simulink model "tp5_5_emetteur_template_usrp"  (R2023a)
settings: Solver=FixedStepDiscrete  StartTime=0.0  StopTime=inf  RelTol=1e-3
PreLoadFcn:
  | T_s_short=160e-6;
  | N=36;
  | N_IFFT=64;
  | T_e = T_s_short/N_IFFT;
  | f_e=1/T_e;
  | 
  | 
  | %% nombre d'éléments nuls à ajouter au vecteur X, resp avant et après les N ss porteuses actives
  | Z_d=ceil((N_IFFT-N)/2);
  | Z_u=floor((N_IFFT-N)/2);
  | 
  | %% taille du préfixe cyclique et temps symbole rallongé
  | v=8;
  | T_s=(N_IFFT+v)*T_e;
  | 
  | %% pilotes
  | r=0.25;
  | 
  | %% la trame
  | t=10;
  | T_t=t*T_s;
  | 
  | %% le codage binaire du message
  | capa_symbole = N*(1-r)*2;
  | str='coucou';
  | message=double(dec2bin(str,8)=='1');% zeros(6-strlength(str),8)];
  | assert(capa_symbole > numel(message), 'message trop long');
  | message_pad=capa_symbole-numel(message);
InitFcn:
  | T_s_short=160e-6;
  | N=36;
  | N_IFFT=64;
  | T_e = T_s_short/N_IFFT;
  | f_e=1/T_e;
  | 
  | 
  | %% nombre d'éléments nuls à ajouter au vecteur X, resp avant et après les N ss porteuses actives
  | Z_d=ceil((N_IFFT-N)/2);
  | Z_u=floor((N_IFFT-N)/2);
  | 
  | %% taille du préfixe cyclique et temps symbole rallongé
  | v=8;
  | T_s=(N_IFFT+v)*T_e;
  | 
  | %% pilotes
  | r=0.25;
  | 
  | %% la trame
  | t=10;
  | T_t=t*T_s;
  | 
  | %% le codage binaire du message
  | capa_symbole = N*(1-r)*2;
  | str='coucou';
  | message=double(dec2bin(str,8)=='1');% zeros(6-strlength(str),8)];
  | assert(capa_symbole > numel(message), 'message trop long');
  | message_pad=capa_symbole-numel(message);
libraries: dspindex x3, commseqgen3 x2, commutil2 x2, commrandsrc3 x1, dspxfrm3 x1, commdigbbndpm3 x1, commsdrhw_v2 x1
Description:
  | This model uses Universal Software Radio Peripheral (USRP) hardware with Simulink(R) to perform FM demodulation and stereo decoding.
settings Model: SimulationMode=accelerator  Creator=speychet  LastModifiedBy=pjoseph
settings SolverCC: AlgebraicLoopSolver=TrustRegion
settings DataIOCC: SaveFormat=Structure  SaveOutput=off  SignalLogging=off  DSMLogging=off  SaveTime=off  ReturnWorkspaceOutputs=off
settings OptimizationCC: ExpressionDepthLimit=2147483647  EfficientMapNaN2IntZero=off  LifeSpan=inf  SimCompilerOptimization=on
settings DebuggingCC: UnderspecifiedInitializationDetection=Classic  MergeDetectMultiDrivingBlocksExec=none  SolverPrmCheckMsg=warning  InheritedTsInSrcMsg=none  MultiTaskCondExecSysMsg=none  ParameterPrecisionLossMsg=none  FcnCallInpInsideContextMsg=warning  UnconnectedInputMsg=warning  UnconnectedOutputMsg=warning  UnconnectedLineMsg=warning  AllowSymbolicDim=off  StateNameClashWarn=warning  SFUnexpectedBacktrackingDiag=warning  SFNoUnconditionalDefaultTransitionDiag=warning  SFExecutionAtInitializationDiag=none  ArithmeticOperatorsInVariantConditions=warning
settings HardwareCC: ProdBitPerPointer=32  ProdBitPerSizeT=32  ProdBitPerPtrDiffT=32  ProdLargestAtomicFloat=None  ProdIntDivRoundTo=Undefined  ProdEndianess=Unspecified  ProdWordSize=32  ProdHWDeviceType=32-bit Generic  TargetBitPerPointer=64  TargetBitPerSizeT=64  TargetBitPerPtrDiffT=64  TargetLongLongMode=on  TargetIntDivRoundTo=Zero  TargetEndianess=LittleEndian  TargetWordSize=64  TargetHWDeviceType=Generic->MATLAB Host Computer  ProdEqTarget=off
settings ModelReferenceCC: EnableRefExpFcnMdlSchedulingChecks=on  PropagateSignalLabelsOutOfModel=off
settings SFSimCC: SimIntegrity=off  SimUseLocalCustomCode=off  CustomCodeUndefinedFunction=UseInterfaceOnly
settings RTWCC: RTWUseLocalCustomCode=off
settings RTWCC: CustomSourceCode=|
  | #include <stdio.h>
  | #include <stdlib.h>
settings CodeAppCC: MaxIdLength=128  StateflowObjectComments=on
settings GRTTargetCC: TargetLangStandard=C89/C90 (ANSI)  CombineOutputUpdateFcns=off  GRTInterface=on
settings ConfigComp: CovMetricSettings=dw  CovSaveCumulativeToWorkspaceVar=on  CovSaveSingleToWorkspaceVar=on  CovExternalEMLEnable=off  CovSFcnEnable=off

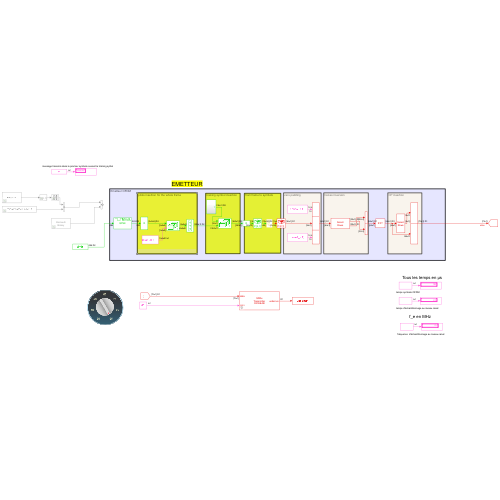
[thumbnail: Simulink's stored preview of the top-level diagram]
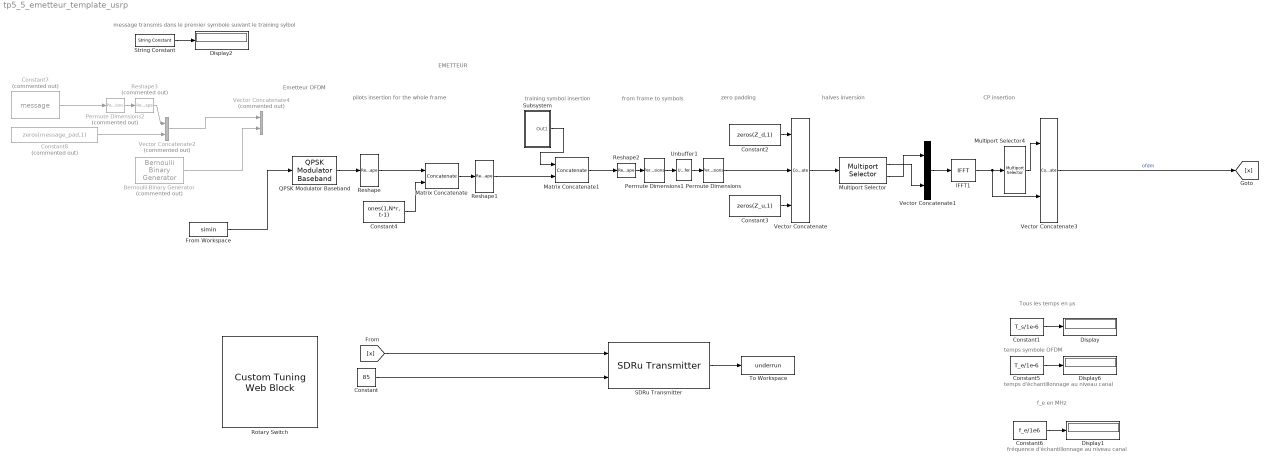
== system tp5_5_emetteur_template_usrp ==
  note: temps symbole OFDM
  note: fréquence d'échantillonnage au niveau canal
  note: CP insertion
  note: temps d'échantillonnage au niveau canal
  note: Tous les temps en µs
  note: pilots insertion for the whole frame
  note: halves inversion
  note: f_e en MHz
  note: zero padding
  note: Emetteur OFDM
  note: EMETTEUR
  note: training symbol insertion
  note: message transmis dans le premier symbole suivant le training sylbol
  note: from frame to symbols
  Bernoulli Binary Generator : commrandsrc3/Bernoulli Binary Generator  Commented=on  ProbabilityOfZero=0.5  SeedSource=Auto  Seed=0  SampleTime=T_t/((t-2)*N*(1-r)*2)  SamplesPerFrame=(t-2)*N*(1-r)*2  OutputDataType=double  SimulateUsing=Code generation
  Constant : Constant  Value=85
  Constant1 : Constant  Value=T_s/1e-6
  Constant2 : Constant  Value=zeros(Z_d,1)
  Constant3 : Constant  Value=zeros(Z_u,1)
  Constant4 : Constant  Value=ones(1,N*r, t-1)  VectorParams1D=off
  Constant5 : Constant  Value=T_e/1e-6
  Constant6 : Constant  Value=f_e/1e6
  Constant7 : Constant  Commented=on  Value=message
  Constant8 : Constant  Commented=on  Value=zeros(message_pad,1)  VectorParams1D=off
  Display{,1..2,6} (4 alike) : Display
  From Workspace : FromWorkspace  VariableName=simin  OutDataTypeStr=double  SampleTime=T_t  Interpolate=off  OutputAfterFinalValue=Holding final value
  IFFT1 : dspxfrm3/IFFT  FFTImplementation=Auto  CompMethod=Table lookup  TableOpt=NEW  TableOptActive=Speed  BitRevOrder=off  cs_in=off  Normalize=on  InheritFFTLength=on  FFTLength=64  WrapInput=on  mode=Complex  outSamplingMode=Sample based  roundingMode=Floor  overflowMode=off  firstCoeffDataTypeStr=Inherit: Same word length as input  firstCoeffLastDataTypeStr=Inherit: Same word length as input  outputMin=[]  outputMax=[]
  Matrix Concatenate : Concatenate  Mode=Multidimensional array
  Matrix Concatenate1 : Concatenate  Mode=Multidimensional array
  Multiport Selector : dspindex/Multiport Selector  rowsOrCols=Rows  idxCellArray={ [1:N_IFFT/2], [N_IFFT/2+1:N_IFFT] }  idxErrMode=Clip Index
  Multiport Selector4 : dspindex/Multiport Selector  rowsOrCols=Rows  idxCellArray={[N_IFFT-v+1:N_IFFT]}  idxErrMode=Clip Index
  Permute Dimensions : PermuteDimensions
  Permute Dimensions1 : PermuteDimensions
  Permute Dimensions2 : PermuteDimensions  Commented=on
  QPSK Modulator Baseband : commdigbbndpm3/QPSK Modulator Baseband  InType=Bit  Enc=Gray  Ph=pi/4  outDtype=double  outWordLen=16  outUDDataType=sfix(16)  outFracLenMode=Best precision  outFracLen=15  outDataTypeStr=double  outLastDataTypeStr=double
  Reshape : Reshape  OutputDimensionality=Customize  OutputDimensions=[(1-r)/r,N*r, t-1]
  Reshape1 : Reshape  OutputDimensionality=Column vector (2-D)
  Reshape2 : Reshape  OutputDimensionality=Customize  OutputDimensions=[N,t]
  Reshape3 : Reshape  Commented=on  OutputDimensionality=Column vector (2-D)
  Rotary Switch : CustomTuningWebBlock  LabelPosition=Hide  ShowInitialText=on  Configuration="{\"components\":[{\"name\":\"RotarySwitchComponent\",\"settings\":{\"arcAngle\":300,\"arcAngleOffset\":120,\"handle\":{\"size\":[150,150],\"src\":\"data:image\\/svg+xml;base64,PHN2ZyBpZD0iTGF5ZXJfMSIgZGF0YS1uYW1lPSJMYXllciAxIiB4bWxucz0iaHR0cDovL3d3dy53My5vcmcvMjAwMC9zdmciIHhtbG5zOnhsaW5rPSJodHRwOi8vd3d3LnczLm9yZy8xOTk5L3hsaW5rIiB2aWV3Qm94PSIwIDAgMTIxIDEyMSI+PGRlZnM+PHN0eWxlPi5jbHMtMXtmaWxsOnVybCgjbGluZWFyLWdyYWRpZW50KTt9LmNscy0yLC5jbHMtM3tmaWxsOiNkMWQxZDE7fS5jbHMtM3tzdHJva2U6I2I3YjdiNztzdHJva2UtbWl0ZXJsaW1pdDoxMDtzdHJva2Utd2lkdGg6MC4yNXB4O30uY2xzLTR7ZmlsbDojZjMwMDAwO30uY2xzLTV7ZmlsbDojZjIxNzY3O308L3N0eWxlPjxsaW5lYXJHcmFkaWVudCBpZD0ibGluZWFyLWdyYWRpZW50IiB4MT0iNjAuNSIgeTE9IjEyMC41IiB4Mj0iNjAuNSIgeTI9IjAuNSIgZ3JhZGllbnRVbml0cz0idXNlclNwYWNlT25Vc2UiPjxzdG9wIG9mZnNldD0iMCIgc3RvcC1jb2xvcj0iI2QxZDFkMSIvPjxzdG9wIG9mZnNldD0iMC4xIiBzdG9wLWNvbG9yPSIjY2VjZWNlIi8+PHN0b3Agb2Zmc2V0PSIwLjE5IiBzdG9wLWNvbG9yPSIjYzNjM2MzIi8+PHN0b3Agb2Zmc2V0PSIwLjI4IiBzdG9wLWNvbG9yPSIjYjFiMWIxIi8+PHN0b3Agb2Zmc2V0PSIwLjM2IiBzdG9wLWNvbG9yPSIjOTg5ODk4Ii8+PHN0b3Agb2Zmc2V0PSIwLjQ0IiBzdG9wLWNvbG9yPSIjNzg3ODc4Ii8+PHN0b3Agb2Zmc2V0PSIwLjQ2IiBzdG9wLWNvbG9yPSIjNmI2YjZiIi8+PHN0b3Agb2Zmc2V0PSIwLjU0IiBzdG9wLWNvbG9yPSIjNmI2YjZiIi8+PHN0b3Agb2Zmc2V0PSIwLjU2IiBzdG9wLWNvbG9yPSIjNzY3Njc2Ii8+PHN0b3Agb2Zmc2V0PSIwLjY0IiBzdG9wLWNvbG9yPSIjOTc5Nzk3Ii8+PHN0b3Agb2Zmc2V0PSIwLjcyIiBzdG9wLWNvbG9yPSIjYjBiMGIwIi8+PHN0b3Agb2Zmc2V0PSIwLjgxIiBzdG9wLWNvbG9yPSIjYzNjM2MzIi8+PHN0b3Agb2Zmc2V0PSIwLjkiIHN0b3AtY29sb3I9IiNjZGNkY2QiLz48c3RvcCBvZmZzZXQ9IjEiIHN0b3AtY29sb3I9IiNkMWQxZDEiLz48L2xpbmVhckdyYWRpZW50PjwvZGVmcz48Y2lyY2xlIGNsYXNzPSJjbHMtMSIgY3g9IjYwLjUiIGN5PSI2MC41IiByPSI2MCIvPjxwYXRoIGNsYXNzPSJjbHMtMiIgZD0iTTYwLjUsMUE1OS41LDU5LjUsMCwxLDEsMSw2MC41LDU5LjU3LDU5LjU3LDAsMCwxLDYwLjUsMW0wLTFBNjAuNSw2MC41LDAsMSwwLDEyMSw2MC41LDYwLjUsNjAuNSwwLDAsMCw2MC41LDBaIi8+PHJlY3QgY2xhc3M9ImNscy0zIiB4PSIwLjUiIHk9IjUxLjUiIHdpZHRoPSIxMjAiIGhlaWdodD0iMTgiIHJ4PSIzLjA0Ii8+PHJlY3QgY2xhc3M9ImNscy00IiB4PSI1Ljc1IiB5PSI1OC43NSIgd2lkdGg9IjE2IiBoZWlnaHQ9IjMiLz48cGF0aCBjbGFzcz0iY2xzLTUiIGQ9Ik0yMS4yNSw1OS4yNXYyaC0xNXYtMmgxNW0xLTFoLTE3djRoMTd2LTRaIi8+PC9zdmc+\"},\"handleOffset\":[0,0],\"handleOrientation\":180,\"handlePosition\":[0,0,1,1],\"handleSize\":{\"height\":0.5,\"width\":0.5},\"labelRadius\":0.36,\"position\":[0,0,1,1],\"states\":[{\"Label\":{\"color\":[0,0,0,1],\"icon\":{\"size\":[0,0],\"src\":[],\"srcOrientation\":\"Right\"},\"iconPlacement\":\"left\",\"opacity\":1,\"position\":[0.7345552884615385,0.6796274038461538],\"show\":true,\"text\":{\"content\":\"30\",\"font\":\"Helvetica\",\"fontSize\":24}},\"Value\":30},{\"Label\":{\"color\":[0,0,0,1],\"icon\":{\"size\":[0,0],\"src\":[],\"srcOrientation\":\"Right\"},\"iconPlacement\":\"left\",\"opacity\":1,\"position\":[0.35757211538461536,0.7603966346153846],\"show\":true,\"text\":{\"content\":\"40\",\"font\":\"Helvetica\",\"fontSize\":24}},\"Value\":40},{\"Label\":{\"color\":[0,0,0,1],\"icon\":{\"size\":[0,0],\"src\":[],\"srcOrientation\":\"Right\"},\"iconPlacement\":\"left\",\"opacity\":1,\"position\":[0.09603365384615385,0.46033653846153844],\"show\":true,\"text\":{\"content\":\"50\",\"font\":\"Helvetica\",\"fontSize\":24}},\"Value\":50},{\"Label\":{\"color\":[0,0,0,1],\"icon\":{\"size\":[0,0],\"src\":[],\"srcOrientation\":\"Right\"},\"iconPlacement\":\"left\",\"opacity\":1,\"position\":[0.36532451923076925,0.1180889423076923],\"show\":true,\"text\":{\"content\":\"60\",\"font\":\"Helvetica\",\"fontSize\":24}},\"Value\":60},{\"Label\":{\"color\":[0,0,0,1],\"icon\":{\"size\":[0,0],\"src\":[],\"srcOrientation\":\"Right\"},\"iconPlacement\":\"left\",\"opacity\":1,\"position\":[0.7191706730769231,0.19501201923076922],\"show\":true,\"text\":{\"content\":\"70\",\"font\":\"Helvetica\",\"fontSize\":24}},\"Value\":70},{\"Label\":{\"color\":[0,0,0,1],\"icon\":{\"size\":[0,0],\"src\":[],\"srcOrientation\":\"Right\"},\"iconPlacement\":\"left\",\"opacity\":1,\"position\":[0.7191706730769231,0.19501201923076922],\"show\":true,\"text\":{\"content\":\"80\",\"font\":\"Helvetica\",\"fontSize\":24}},\"Value\":80},{\"Label\":{\"color\":[0,0,0,1],\"icon\":{\"size\":[0,0],\"src\":[],\"srcOrientation\":\"Right\"},\"iconPlacement\":\"left\",\"opacity\":1,\"position\":[0.7191706730769231,0.19501201923076922],\"show\":true,\"text\":{\"content\":\"85\",\"font\":\"Helvetica\",\"fontSize\":24}},\"Value\":85}],\"tickRadius\":0.32}},{\"name\":\"BackgroundImageComponent\",\"settings\":{\"image\":{\"size\":[155,150],\"src\":\"data:image\\/svg+xml;base64,PD94bWwgdmVyc2lvbj0iMS4wIiBlbmNvZGluZz0idXRmLTgiPz4NCjwhLS0gR2VuZXJhdG9yOiBBZG9iZSBJbGx1c3RyYXRvciAyNS4wLjAsIFNWRyBFeHBvcnQgUGx1Zy1JbiAuIFNWRyBWZXJzaW9uOiA2LjAwIEJ1aWxkIDApICAtLT4NCjxzdmcgdmVyc2lvbj0iMS4xIg0KCSBpZD0iTGF5ZXJfMl8xXyIgeG1sbnM6Y2M9Imh0dHA6Ly9jcmVhdGl2ZWNvbW1vbnMub3JnL25zIyIgeG1sbnM6ZGM9Imh0dHA6Ly9wdXJsLm9yZy9kYy9lbGVtZW50cy8xLjEvIiB4bWxuczppbmtzY2FwZT0iaHR0cDovL3d3dy5pbmtzY2FwZS5vcmcv ...(+4184 chars)\",\"srcOrientation\":\"Right\"},\"position\":[0,0,1,1],\"scaleMode\":\"0\"}},{\"name\":\"ForegroundImageComponent\",\"settings\":{\"image\":{\"size\":[0,0],\"src\":\"default\",\"srcOrientation\":[]},\"isForeground\":1,\"position\":[0,0,1,1],\"scaleMode\":\"0\"}}],\"settings\":{\"BindingType\":\"param\",\"backgroundColor\":[0,0,255,\"1\"],\"backgroundOffset\":1,\"fixedAspectRatio\":\"on\",\"image\":{\"size\":[150,150],\"src\":\"data:image\\/svg+xml;base64,PD94bWwgdmVyc2lvbj0iMS4wIiBlbmNvZGluZz0iVVRGLTgiIHN0YW5kYWxvbmU9Im5vIj8+CjwhLS0gR2VuZXJhdG9yOiBBZG9iZSBJbGx1c3RyYXRvciAxOS4yLjEsIFNWRyBFeHBvcnQgUGx1Zy1JbiAuIFNWRyBWZXJzaW9uOiA2LjAwIEJ1aWxkIDApICAtLT4KCjxzdmcKICAgeG1sbnM6ZGM9Imh0dHA6Ly9wdXJsLm9yZy9kYy9lbGVtZW50cy8xLjEvIgogICB4bWxuczpjYz0iaHR0cDovL2NyZWF0aXZlY29tbW9ucy5vcmcvbnMjIgogICB4bWxuczpyZGY9Imh0dHA6Ly93d3cudzMub3JnLzE5OTkvMDIvMjItcmRmLXN5bnRh ...(+9660 chars)\"},\"showBackgroundColor\":false,\"variant\":\"rotarySwitch\",\"version\":\"R2022a\"},\"type\":\"RotarySwitch\"}"
  SDRu Transmitter : commsdrhw_v2/SDRu Transmitter  rxtx=tx  initializeIPAddress=0  devMap=0  USRP2_IP=192.168.10.2  USRP_IP_X300=192.168.10.2  USRP_IP_X310=192.168.10.2  USRP_IP_N300=No devices found  USRP_IP_N310=192.168.10.2  USRP_IP_N320=No devices found  USRP_serialNumB200=3136D21  USRP_serialNumB210=30CEEAB  platform=B210  prevPlatform=B210  lastIPAddressPopup=192.168.10.2  USRP_ID=30CEEAB  LastIPAddress=192.168.10.2  ChannelMapping=1  centerFrequencySrc=Dialog  centerFrequency=433.5e6  loOffsetSrc=Dialog  loOffset=200e3  gainSrc=Input port  gain=8  PPSSource=Internal  EnableGPSLock=off  EnsureSyncGPSTime=off  clockSource=Internal  EnableRefLock=off  masterClkRateParam=8000000  masterClkRateB200=32e6  masterClkRateB210=f_e*20  masterClkRateX300=200e6  masterClkRateX310=200e6  masterClkRateN300=125e6  masterClkRateN310=125e6  masterClkRateN320=200e6  decimInterpSrc=Dialog  lastDecimSource=Dialog  decimInterp=20  USRP2_IP_NUM=[51 48 67 69 69 65 66]  frameLength=362  sampleRate=399999.99999999994  TransportDataType=int16  outputDatatype=Same as transport data type  overrunUnderrunPort=on  sampleTime=5.12e-06  dboardInfo=|  HOST_DATA_PORT=30000  HOST_CONTROL_PORT=30001  USRP2_DATA_PORT=32769  USRP2_CONTROL_PORT=32768  bufferMode=Continuous streaming  EnableBurstMode=off  NumFramesInBurst=100
      | dbid: 0
      |           dbName: 'no db found'
      |          freqMin: 0
      |          freqMax: 0
      |          gainMin: 0
      |          gainMax: 0
      |     gainStepSize: 0
  String Constant : StringConstant  String=str
  Subsystem : Subsystem
  To Workspace : ToWorkspace  VariableName=underrun  SaveFormat=Timeseries  SampleTime=-1
      settings: MaxDataPoints=4e5
  Unbuffer1 : Unbuffer
  Vector Concatenate : Concatenate  NumInputs=3
  Vector Concatenate1 : Concatenate
  Vector Concatenate2 : Concatenate  Commented=on
  Vector Concatenate3 : Concatenate
  Vector Concatenate4 : Concatenate  Commented=on
  wires:
  Constant3/1 -> Vector Concatenate/3
  Constant1/1 -> Display/1
  Constant5/1 -> Display6/1
  Constant2/1 -> Vector Concatenate/1
  Constant4/1 -> Matrix Concatenate/2
  Vector Concatenate/1 -> Multiport Selector/1
  Matrix Concatenate/1 -> Reshape1/1
  Multiport Selector4/1 -> Vector Concatenate3/1
  QPSK Modulator Baseband/1 -> Reshape/1
  Multiport Selector/1 -> Vector Concatenate1/2
  Reshape/1 -> Matrix Concatenate/1
  Unbuffer1/1 -> Permute Dimensions/1
  IFFT1/1 -> Multiport Selector4/1, Vector Concatenate3/2
  Subsystem/1(Out1) -> Matrix Concatenate1/1
  Matrix Concatenate1/1 -> Reshape2/1
  Permute Dimensions1/1 -> Unbuffer1/1
  Vector Concatenate1/1 -> IFFT1/1
  Reshape1/1 -> Matrix Concatenate1/2
  Bernoulli Binary Generator/1 -> Vector Concatenate4/2
  Constant6/1 -> Display1/1
  Reshape2/1 -> Permute Dimensions1/1
  Multiport Selector/2 -> Vector Concatenate1/1
  Vector Concatenate3/1 -> [x]  "ofdm"
  Permute Dimensions/1 -> Vector Concatenate/2
  Constant/1 -> SDRu Transmitter/2
  Permute Dimensions2/1 -> Reshape3/1
  String Constant/1 -> Display2/1
  Vector Concatenate2/1 -> Vector Concatenate4/1
  Constant8/1 -> Vector Concatenate2/2
  Reshape3/1 -> Vector Concatenate2/1
  Constant7/1 -> Permute Dimensions2/1
  SDRu Transmitter/1 -> To Workspace/1
  [x] -> SDRu Transmitter/1
  From Workspace/1 -> QPSK Modulator Baseband/1

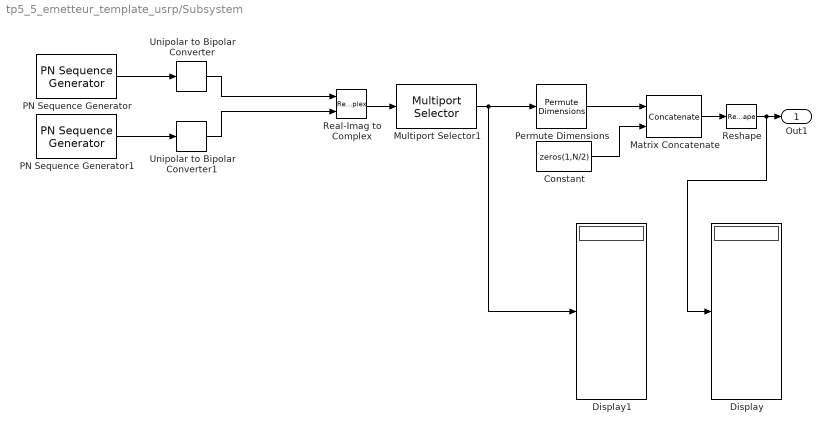
== system tp5_5_emetteur_template_usrp/Subsystem ==
  Constant : Constant  Value=zeros(1,N/2)  VectorParams1D=off
  Display : Display
  Display1 : Display
  Matrix Concatenate : Concatenate  Mode=Multidimensional array
  Multiport Selector1 : dspindex/Multiport Selector  rowsOrCols=Rows  idxCellArray=1:N/2  idxErrMode=Clip Index
  PN Sequence Generator : commseqgen3/PN Sequence Generator  poly='z^6 + z + 1'  ini_sta=[0 0 0 0 0 1]  outBitMaskSource=Dialog parameter  shift=0  outVarSiz=off  maxOutSizeMode=Dialog parameter  maxOutSize=[10 1]  Ts=T_t/63  sampPerFrame=63  reset=off  bitPackedOutputs=off  outDataType=double  numPackedBits=8  bitPackDataSigned=off  bitPackedOutDType=double
  PN Sequence Generator1 : commseqgen3/PN Sequence Generator  poly='z^6 + z + 1'  ini_sta=[1 0 0 0 0 1]  outBitMaskSource=Dialog parameter  shift=0  outVarSiz=off  maxOutSizeMode=Dialog parameter  maxOutSize=[10 1]  Ts=T_t/63  sampPerFrame=63  reset=off  bitPackedOutputs=off  outDataType=double  numPackedBits=8  bitPackDataSigned=off  bitPackedOutDType=double
  Permute Dimensions : PermuteDimensions
  Real-Imag to Complex : RealImagToComplex
  Reshape : Reshape  OutputDimensionality=Column vector (2-D)
  Unipolar to Bipolar Converter : commutil2/Unipolar to Bipolar Converter  M=2  polarity=Positive  dataType=Inherit via internal rule
  Unipolar to Bipolar Converter1 : commutil2/Unipolar to Bipolar Converter  M=2  polarity=Positive  dataType=Inherit via internal rule
  Out1 : Outport
  wires:
  PN Sequence Generator1/1 -> Unipolar to Bipolar Converter1/1
  PN Sequence Generator/1 -> Unipolar to Bipolar Converter/1
  Real-Imag to Complex/1 -> Multiport Selector1/1
  Multiport Selector1/1 -> Permute Dimensions/1, Display1/1
  Permute Dimensions/1 -> Matrix Concatenate/1
  Matrix Concatenate/1 -> Reshape/1
  Constant/1 -> Matrix Concatenate/2
  Reshape/1 -> Display/1, Out1/1
  Unipolar to Bipolar Converter/1 -> Real-Imag to Complex/1
  Unipolar to Bipolar Converter1/1 -> Real-Imag to Complex/2
